simulink model "SIFT-save"  (R2016a)
settings: Solver=VariableStepAuto  StartTime=0.0  StopTime=10.0  RelTol=1e-3
libraries: visionhdlfilter x4, visionhdlio x2, visionsources x1, visiongeotforms x1
settings Model: Creator=Gururaja  LastModifiedBy=Gururaja

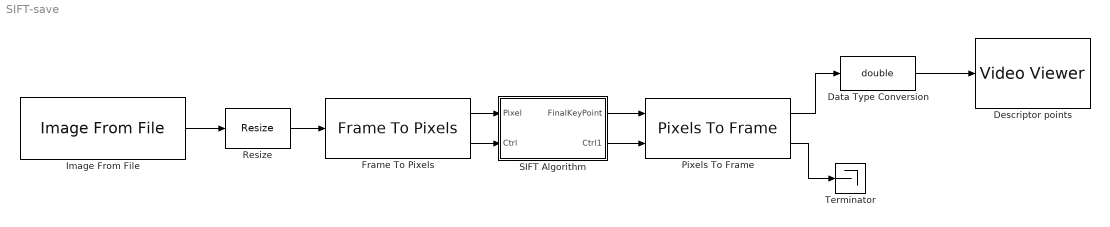
== system SIFT-save ==
  Data Type Conversion : DataTypeConversion  OutDataTypeStr=double
  Descriptor points : VideoViewer
  Frame To Pixels : visionhdlio/Frame To Pixels  NumComponents=1  VideoFormat=1080p  ActivePixelsPerLine=32  ActiveVideoLines=18  TotalPixelsPerLine=42  TotalVideoLines=28  StartingActiveLine=6  FrontPorch=5  SampleTime=0
  Image From File : visionsources/Image From File  Tag=vipblks_nd  FileName=peppers.png  imagePorts=One multidimensional signal  Ts=inf  ImageDataType=Inherit from input image  Signed=on  WordLength=16  sdImageDataType=uint(8)  FractionLengthMode=User-defined  FractionLength=15  OutPortLabels=R|G|B
  Pixels To Frame : visionhdlio/Pixels To Frame  NumComponents=1  VideoFormat=1080p  ActivePixelsPerLine=32  ActiveVideoLines=18  TotalPixelsPerLine=42  TotalVideoLines=28
  Resize : visiongeotforms/Resize  specify=Output size as a percentage of input size  rfactor=[200 150]  outCols=25  outRows=25  outRowsCols=[25 35]  interp_method=Bilinear  antialias=on  useROI=off  roiFlag=off  prodOutputMode=Binary point scaling  prodOutputWordLength=32  prodOutputFracLength=10  roundingMode=Nearest  overflowMode=on
  SIFT Algorithm : Subsystem
  Terminator : Terminator
  wires:
  Image From File/1 -> Resize/1
  Resize/1 -> Frame To Pixels/1
  Frame To Pixels/1 -> SIFT Algorithm/1(Pixel)
  Frame To Pixels/2 -> SIFT Algorithm/2(Ctrl)
  SIFT Algorithm/1(FinalKeyPoint) -> Pixels To Frame/1
  SIFT Algorithm/2(Ctrl1) -> Pixels To Frame/2
  Pixels To Frame/2 -> Terminator/1
  Pixels To Frame/1 -> Data Type Conversion/1
  Data Type Conversion/1 -> Descriptor points/1

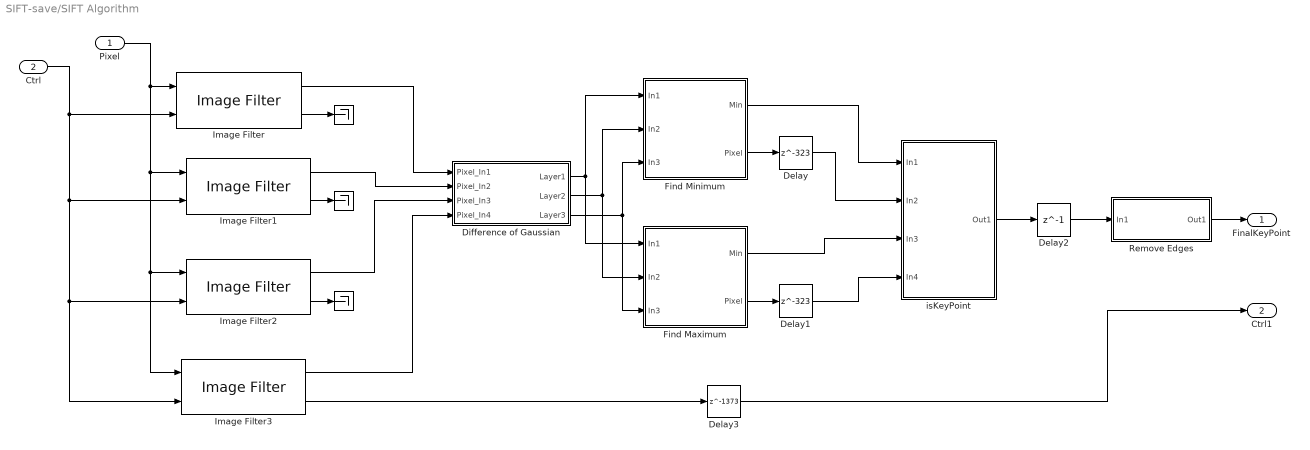
== system SIFT-save/SIFT Algorithm ==
  Pixel : Inport
  Ctrl : Inport  Port=2
  " " : Terminator
  " " : Terminator
  " " : Terminator
  Delay : Delay  DelayLength=323  InitialCondition=0
  Delay1 : Delay  DelayLength=323  InitialCondition=0
  Delay2 : Delay  DelayLength=1  InitialCondition=0
  Delay3 : Delay  DelayLength=1373  InitialCondition=0
  Difference of Gaussian : Subsystem
  Find Maximum : Subsystem
  Find Minimum : Subsystem
  Image Filter{,1..3} (4 alike) : visionhdlfilter/Image Filter  Coefficients=[ 1, 0; 0, -1 ]  PaddingMethod=Constant  PaddingValue=0  LineBufferSize=2048  roundingMode=Floor  overflowMode=off  CoeffMin=[]  CoeffMax=[]  OutputMin=[]  OutputMax=[]  SimulateUsing=Code generation
  Remove Edges : Subsystem
  isKeyPoint : Subsystem
  FinalKeyPoint : Outport
  Ctrl1 : Outport  Port=2
  wires:
  Pixel/1 -> Image Filter/1, Image Filter1/1, Image Filter3/1, Image Filter2/1
  Ctrl/1 -> Image Filter/2, Image Filter1/2, Image Filter2/2, Image Filter3/2
  Image Filter2/2 -> " "/1
  Image Filter1/2 -> " "/1
  Image Filter/2 -> " "/1
  Image Filter/1 -> Difference of Gaussian/1(Pixel_In1)
  Image Filter1/1 -> Difference of Gaussian/2(Pixel_In2)
  Image Filter2/1 -> Difference of Gaussian/3(Pixel_In3)
  Image Filter3/1 -> Difference of Gaussian/4(Pixel_In4)
  Difference of Gaussian/1(Layer1) -> Find Maximum/1(In1), Find Minimum/1(In1)
  Difference of Gaussian/2(Layer2) -> Find Maximum/2(In2), Find Minimum/2(In2)
  Difference of Gaussian/3(Layer3) -> Find Maximum/3(In3), Find Minimum/3(In3)
  Find Minimum/2(Pixel) -> Delay/1
  Find Minimum/1(Min) -> isKeyPoint/1(In1)
  Delay/1 -> isKeyPoint/2(In2)
  Delay1/1 -> isKeyPoint/4(In4)
  isKeyPoint/1(Out1) -> Delay2/1
  Delay2/1 -> Remove Edges/1(In1)
  Remove Edges/1(Out1) -> FinalKeyPoint/1
  Image Filter3/2 -> Delay3/1
  Delay3/1 -> Ctrl1/1
  Find Maximum/1(Min) -> isKeyPoint/3(In3)
  Find Maximum/2(Pixel) -> Delay1/1

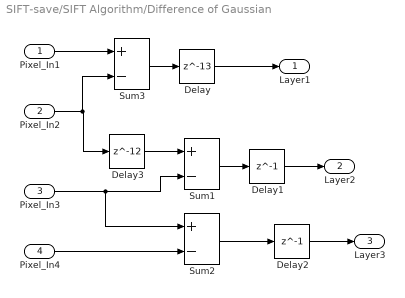
== system SIFT-save/SIFT Algorithm/Difference of Gaussian ==
  Pixel_In1 : Inport
  Pixel_In2 : Inport  Port=2
  Pixel_In3 : Inport  Port=3
  Pixel_In4 : Inport  Port=4
  Delay : Delay  DelayLength=13  InitialCondition=0
  Delay1 : Delay  DelayLength=1  InitialCondition=0
  Delay2 : Delay  DelayLength=1  InitialCondition=0
  Delay3 : Delay  DelayLength=12  InitialCondition=0
  Sum1 : Sum  Inputs=+-
  Sum2 : Sum  Inputs=+-
  Sum3 : Sum  Inputs=+-
  Layer1 : Outport
  Layer2 : Outport  Port=2
  Layer3 : Outport  Port=3
  wires:
  Pixel_In1/1 -> Sum3/1
  Pixel_In2/1 -> Sum3/2, Delay3/1
  Delay3/1 -> Sum1/1
  Pixel_In3/1 -> Sum2/1, Sum1/2
  Pixel_In4/1 -> Sum2/2
  Sum3/1 -> Delay/1
  Sum1/1 -> Delay1/1
  Sum2/1 -> Delay2/1
  Delay2/1 -> Layer3/1
  Delay1/1 -> Layer2/1
  Delay/1 -> Layer1/1

== system SIFT-save/SIFT Algorithm/Find Maximum ==
  In1 : Inport
  In2 : Inport  Port=2
  In3 : Inport  Port=3
  Min/Max DOG1 : Subsystem
  Min/Max DOG2 : Subsystem
  Min/Max DOG3 : Subsystem
  MinMax : MinMax  Function=max  Inputs=26
  Min : Outport
  Pixel : Outport  Port=2
  wires:
  In2/1 -> Min/Max DOG1/1(In1)
  Min/Max DOG1/5(Out5) -> Pixel/1
  Min/Max DOG2/1(Out1) -> MinMax/18
  Min/Max DOG2/9(Out9) -> MinMax/26
  Min/Max DOG2/2(Out2) -> MinMax/19
  Min/Max DOG2/3(Out3) -> MinMax/20
  Min/Max DOG2/4(Out4) -> MinMax/21
  Min/Max DOG2/5(Out5) -> MinMax/22
  Min/Max DOG2/6(Out6) -> MinMax/23
  Min/Max DOG2/7(Out7) -> MinMax/24
  Min/Max DOG2/8(Out8) -> MinMax/25
  Min/Max DOG3/1(Out1) -> MinMax/1
  Min/Max DOG3/3(Out3) -> MinMax/3
  Min/Max DOG3/2(Out2) -> MinMax/2
  Min/Max DOG3/4(Out4) -> MinMax/4
  Min/Max DOG3/5(Out5) -> MinMax/5
  Min/Max DOG3/6(Out6) -> MinMax/6
  Min/Max DOG3/7(Out7) -> MinMax/7
  Min/Max DOG3/8(Out8) -> MinMax/8
  Min/Max DOG3/9(Out9) -> MinMax/9
  MinMax/1 -> Min/1
  Min/Max DOG1/1(Out1) -> MinMax/10
  Min/Max DOG1/2(Out2) -> MinMax/11
  Min/Max DOG1/3(Out3) -> MinMax/12
  Min/Max DOG1/4(Out4) -> MinMax/13
  Min/Max DOG1/6(Out6) -> MinMax/14
  Min/Max DOG1/7(Out7) -> MinMax/15
  Min/Max DOG1/8(Out8) -> MinMax/16
  Min/Max DOG1/9(Out9) -> MinMax/17
  In1/1 -> Min/Max DOG3/1(In1)
  In3/1 -> Min/Max DOG2/1(In1)

== system SIFT-save/SIFT Algorithm/Find Minimum ==
  In1 : Inport
  In2 : Inport  Port=2
  In3 : Inport  Port=3
  Min/Max DOG1 : Subsystem
  Min/Max DOG2 : Subsystem
  Min/Max DOG3 : Subsystem
  MinMax : MinMax  Inputs=26
  Min : Outport
  Pixel : Outport  Port=2
  wires:
  In2/1 -> Min/Max DOG1/1(In1)
  Min/Max DOG1/5(Out5) -> Pixel/1
  Min/Max DOG2/1(Out1) -> MinMax/18
  Min/Max DOG2/9(Out9) -> MinMax/26
  Min/Max DOG2/2(Out2) -> MinMax/19
  Min/Max DOG2/3(Out3) -> MinMax/20
  Min/Max DOG2/4(Out4) -> MinMax/21
  Min/Max DOG2/5(Out5) -> MinMax/22
  Min/Max DOG2/6(Out6) -> MinMax/23
  Min/Max DOG2/7(Out7) -> MinMax/24
  Min/Max DOG2/8(Out8) -> MinMax/25
  Min/Max DOG3/1(Out1) -> MinMax/1
  Min/Max DOG3/3(Out3) -> MinMax/3
  Min/Max DOG3/2(Out2) -> MinMax/2
  Min/Max DOG3/4(Out4) -> MinMax/4
  Min/Max DOG3/5(Out5) -> MinMax/5
  Min/Max DOG3/6(Out6) -> MinMax/6
  Min/Max DOG3/7(Out7) -> MinMax/7
  Min/Max DOG3/8(Out8) -> MinMax/8
  Min/Max DOG3/9(Out9) -> MinMax/9
  MinMax/1 -> Min/1
  Min/Max DOG1/1(Out1) -> MinMax/10
  Min/Max DOG1/2(Out2) -> MinMax/11
  Min/Max DOG1/3(Out3) -> MinMax/12
  Min/Max DOG1/4(Out4) -> MinMax/13
  Min/Max DOG1/6(Out6) -> MinMax/14
  Min/Max DOG1/7(Out7) -> MinMax/15
  Min/Max DOG1/8(Out8) -> MinMax/16
  Min/Max DOG1/9(Out9) -> MinMax/17
  In1/1 -> Min/Max DOG3/1(In1)
  In3/1 -> Min/Max DOG2/1(In1)

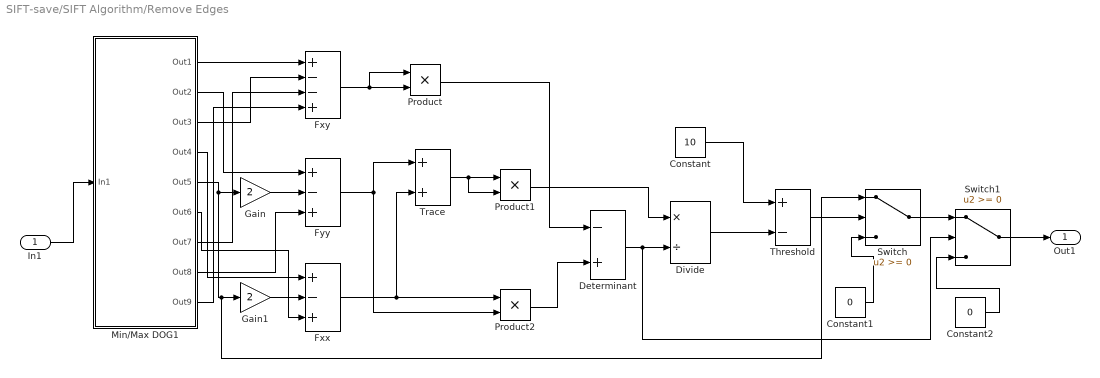
== system SIFT-save/SIFT Algorithm/Remove Edges ==
  In1 : Inport
  Constant : Constant  Value=10
  Constant1 : Constant  Value=0
  Constant2 : Constant  Value=0
  Determinant : Sum  Inputs=-+
  Divide : Product  Inputs=*/
  Fxx : Sum  Inputs=+-+
  Fxy : Sum  Inputs=+--+
  Fyy : Sum  Inputs=+-+
  Gain : Gain  Gain=2
  Gain1 : Gain  Gain=2
  Min/Max DOG1 : Subsystem
  Product : Product
  Product1 : Product
  Product2 : Product
  Switch : Switch
  Switch1 : Switch
  Threshold : Sum  Inputs=+-
  Trace : Sum
  Out1 : Outport
  wires:
  In1/1 -> Min/Max DOG1/1(In1)
  Min/Max DOG1/1(Out1) -> Fxy/1
  Min/Max DOG1/3(Out3) -> Fxy/2
  Gain1/1 -> Fxx/2
  Gain/1 -> Fyy/2
  Min/Max DOG1/2(Out2) -> Fyy/1
  Min/Max DOG1/4(Out4) -> Fxx/1
  Min/Max DOG1/6(Out6) -> Fxx/3
  Min/Max DOG1/7(Out7) -> Fxy/3
  Min/Max DOG1/8(Out8) -> Fyy/3
  Min/Max DOG1/9(Out9) -> Fxy/4
  Fyy/1 -> Product2/2, Trace/1
  Fxy/1 -> Product/1, Product/2
  Trace/1 -> Product1/2, Product1/1
  Fxx/1 -> Trace/2, Product2/1
  Product2/1 -> Determinant/2
  Product/1 -> Determinant/1
  Determinant/1 -> Switch1/2, Divide/2
  Product1/1 -> Divide/1
  Divide/1 -> Threshold/2
  Constant/1 -> Threshold/1
  Threshold/1 -> Switch/2
  Constant1/1 -> Switch/3
  Min/Max DOG1/5(Out5) -> Switch/1, Gain1/1, Gain/1
  Switch/1 -> Switch1/1
  Constant2/1 -> Switch1/3
  Switch1/1 -> Out1/1

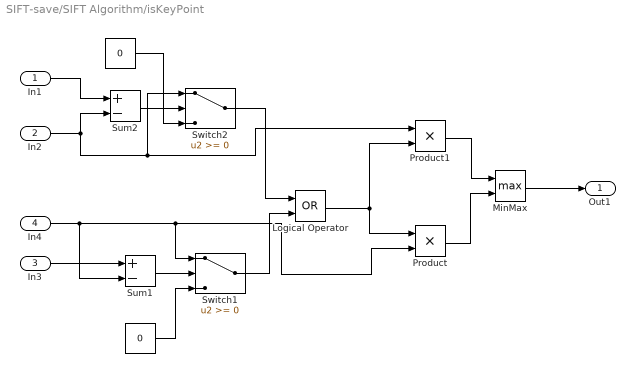
== system SIFT-save/SIFT Algorithm/isKeyPoint ==
  In1 : Inport
  In2 : Inport  Port=2
  In3 : Inport  Port=3
  In4 : Inport  Port=4
  " " : Constant  Value=0
  " " : Constant  Value=0
  Logical Operator : Logic  Operator=OR  AllPortsSameDT=off  OutDataTypeStr=boolean
  MinMax : MinMax  Function=max  Inputs=2
  Product : Product
  Product1 : Product
  Sum1 : Sum  Inputs=+-
  Sum2 : Sum  Inputs=+-
  Switch1 : Switch
  Switch2 : Switch
  Out1 : Outport
  wires:
  In1/1 -> Sum2/1
  In2/1 -> Sum2/2, Switch2/1, Product1/1
  Sum1/1 -> Switch1/2
  Sum2/1 -> Switch2/2
  " "/1 -> Switch2/3
  " "/1 -> Switch1/3
  In3/1 -> Sum1/1
  Switch2/1 -> Logical Operator/1
  Switch1/1 -> Logical Operator/2
  Product1/1 -> MinMax/1
  Product/1 -> MinMax/2
  MinMax/1 -> Out1/1
  Logical Operator/1 -> Product1/2, Product/1
  In4/1 -> Sum1/2, Switch1/1, Product/2

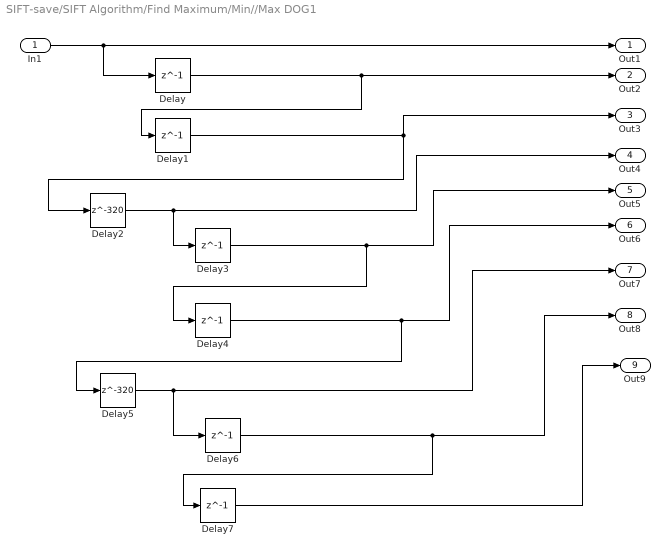
== system SIFT-save/SIFT Algorithm/Find Maximum/Min//Max DOG1 ==
  In1 : Inport
  Delay{,1,3..4,6..7} (6 alike) : Delay  DelayLength=1  InitialCondition=0
  Delay2 : Delay  DelayLength=320  InitialCondition=0
  Delay5 : Delay  DelayLength=320  InitialCondition=0
  Out1 : Outport
  Out2 : Outport  Port=2
  Out3 : Outport  Port=3
  Out4 : Outport  Port=4
  Out5 : Outport  Port=5
  Out6 : Outport  Port=6
  Out7 : Outport  Port=7
  Out8 : Outport  Port=8
  Out9 : Outport  Port=9
  wires:
  In1/1 -> Delay/1, Out1/1
  Delay/1 -> Out2/1, Delay1/1
  Delay1/1 -> Out3/1, Delay2/1
  Delay2/1 -> Delay3/1, Out4/1
  Delay3/1 -> Delay4/1, Out5/1
  Delay4/1 -> Delay5/1, Out6/1
  Delay5/1 -> Delay6/1, Out7/1
  Delay6/1 -> Delay7/1, Out8/1
  Delay7/1 -> Out9/1

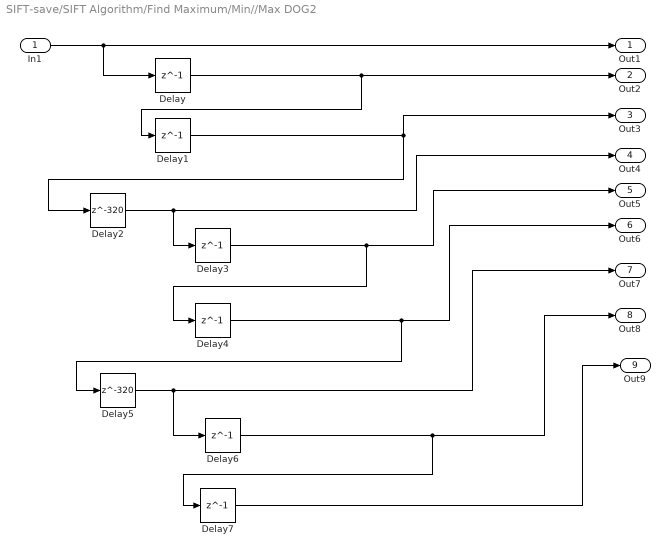
== system SIFT-save/SIFT Algorithm/Find Maximum/Min//Max DOG2 ==
  In1 : Inport
  Delay{,1,3..4,6..7} (6 alike) : Delay  DelayLength=1  InitialCondition=0
  Delay2 : Delay  DelayLength=320  InitialCondition=0
  Delay5 : Delay  DelayLength=320  InitialCondition=0
  Out1 : Outport
  Out2 : Outport  Port=2
  Out3 : Outport  Port=3
  Out4 : Outport  Port=4
  Out5 : Outport  Port=5
  Out6 : Outport  Port=6
  Out7 : Outport  Port=7
  Out8 : Outport  Port=8
  Out9 : Outport  Port=9
  wires:
  In1/1 -> Delay/1, Out1/1
  Delay/1 -> Out2/1, Delay1/1
  Delay1/1 -> Out3/1, Delay2/1
  Delay2/1 -> Delay3/1, Out4/1
  Delay3/1 -> Delay4/1, Out5/1
  Delay4/1 -> Delay5/1, Out6/1
  Delay5/1 -> Delay6/1, Out7/1
  Delay6/1 -> Delay7/1, Out8/1
  Delay7/1 -> Out9/1

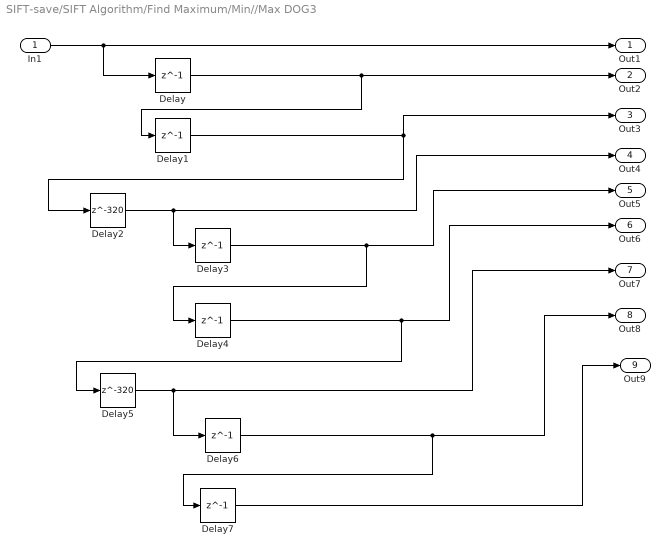
== system SIFT-save/SIFT Algorithm/Find Maximum/Min//Max DOG3 ==
  In1 : Inport
  Delay{,1,3..4,6..7} (6 alike) : Delay  DelayLength=1  InitialCondition=0
  Delay2 : Delay  DelayLength=320  InitialCondition=0
  Delay5 : Delay  DelayLength=320  InitialCondition=0
  Out1 : Outport
  Out2 : Outport  Port=2
  Out3 : Outport  Port=3
  Out4 : Outport  Port=4
  Out5 : Outport  Port=5
  Out6 : Outport  Port=6
  Out7 : Outport  Port=7
  Out8 : Outport  Port=8
  Out9 : Outport  Port=9
  wires:
  In1/1 -> Delay/1, Out1/1
  Delay/1 -> Out2/1, Delay1/1
  Delay1/1 -> Out3/1, Delay2/1
  Delay2/1 -> Delay3/1, Out4/1
  Delay3/1 -> Delay4/1, Out5/1
  Delay4/1 -> Delay5/1, Out6/1
  Delay5/1 -> Delay6/1, Out7/1
  Delay6/1 -> Delay7/1, Out8/1
  Delay7/1 -> Out9/1

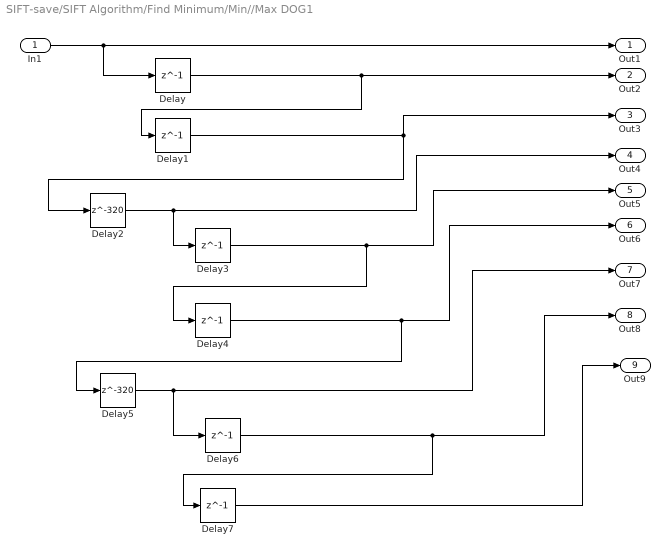
== system SIFT-save/SIFT Algorithm/Find Minimum/Min//Max DOG1 ==
  In1 : Inport
  Delay{,1,3..4,6..7} (6 alike) : Delay  DelayLength=1  InitialCondition=0
  Delay2 : Delay  DelayLength=320  InitialCondition=0
  Delay5 : Delay  DelayLength=320  InitialCondition=0
  Out1 : Outport
  Out2 : Outport  Port=2
  Out3 : Outport  Port=3
  Out4 : Outport  Port=4
  Out5 : Outport  Port=5
  Out6 : Outport  Port=6
  Out7 : Outport  Port=7
  Out8 : Outport  Port=8
  Out9 : Outport  Port=9
  wires:
  In1/1 -> Delay/1, Out1/1
  Delay/1 -> Out2/1, Delay1/1
  Delay1/1 -> Out3/1, Delay2/1
  Delay2/1 -> Delay3/1, Out4/1
  Delay3/1 -> Delay4/1, Out5/1
  Delay4/1 -> Delay5/1, Out6/1
  Delay5/1 -> Delay6/1, Out7/1
  Delay6/1 -> Delay7/1, Out8/1
  Delay7/1 -> Out9/1

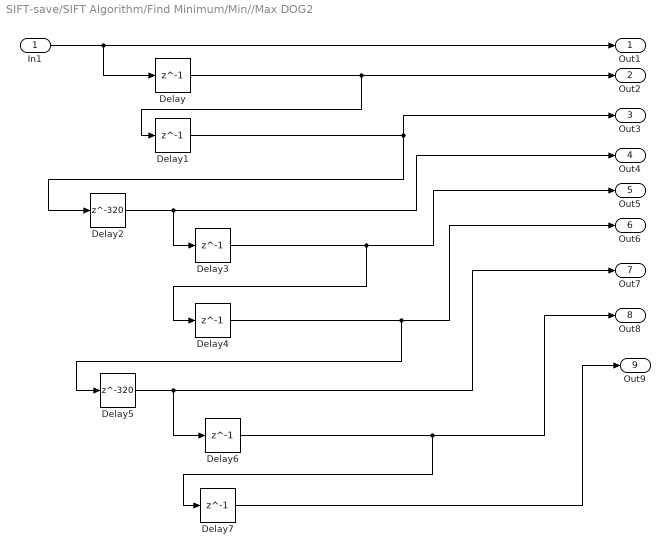
== system SIFT-save/SIFT Algorithm/Find Minimum/Min//Max DOG2 ==
  In1 : Inport
  Delay{,1,3..4,6..7} (6 alike) : Delay  DelayLength=1  InitialCondition=0
  Delay2 : Delay  DelayLength=320  InitialCondition=0
  Delay5 : Delay  DelayLength=320  InitialCondition=0
  Out1 : Outport
  Out2 : Outport  Port=2
  Out3 : Outport  Port=3
  Out4 : Outport  Port=4
  Out5 : Outport  Port=5
  Out6 : Outport  Port=6
  Out7 : Outport  Port=7
  Out8 : Outport  Port=8
  Out9 : Outport  Port=9
  wires:
  In1/1 -> Delay/1, Out1/1
  Delay/1 -> Out2/1, Delay1/1
  Delay1/1 -> Out3/1, Delay2/1
  Delay2/1 -> Delay3/1, Out4/1
  Delay3/1 -> Delay4/1, Out5/1
  Delay4/1 -> Delay5/1, Out6/1
  Delay5/1 -> Delay6/1, Out7/1
  Delay6/1 -> Delay7/1, Out8/1
  Delay7/1 -> Out9/1

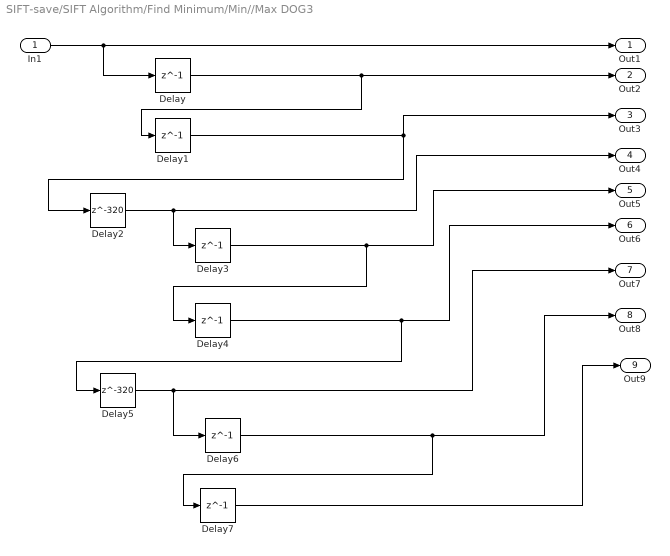
== system SIFT-save/SIFT Algorithm/Find Minimum/Min//Max DOG3 ==
  In1 : Inport
  Delay{,1,3..4,6..7} (6 alike) : Delay  DelayLength=1  InitialCondition=0
  Delay2 : Delay  DelayLength=320  InitialCondition=0
  Delay5 : Delay  DelayLength=320  InitialCondition=0
  Out1 : Outport
  Out2 : Outport  Port=2
  Out3 : Outport  Port=3
  Out4 : Outport  Port=4
  Out5 : Outport  Port=5
  Out6 : Outport  Port=6
  Out7 : Outport  Port=7
  Out8 : Outport  Port=8
  Out9 : Outport  Port=9
  wires:
  In1/1 -> Delay/1, Out1/1
  Delay/1 -> Out2/1, Delay1/1
  Delay1/1 -> Out3/1, Delay2/1
  Delay2/1 -> Delay3/1, Out4/1
  Delay3/1 -> Delay4/1, Out5/1
  Delay4/1 -> Delay5/1, Out6/1
  Delay5/1 -> Delay6/1, Out7/1
  Delay6/1 -> Delay7/1, Out8/1
  Delay7/1 -> Out9/1

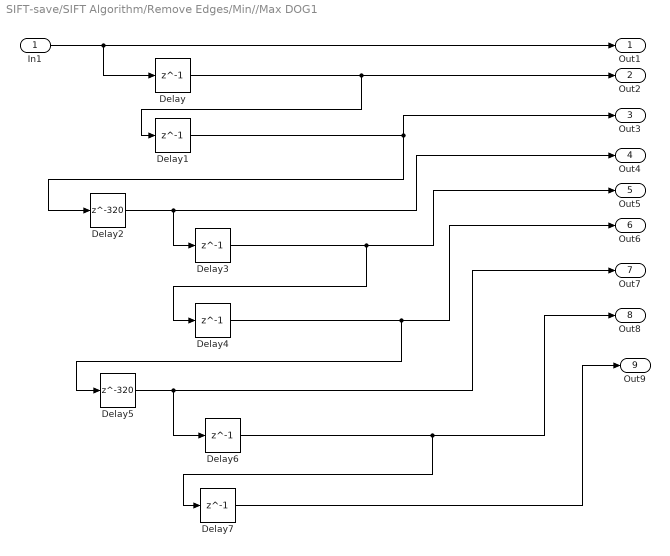
== system SIFT-save/SIFT Algorithm/Remove Edges/Min//Max DOG1 ==
  In1 : Inport
  Delay{,1,3..4,6..7} (6 alike) : Delay  DelayLength=1  InitialCondition=0
  Delay2 : Delay  DelayLength=320  InitialCondition=0
  Delay5 : Delay  DelayLength=320  InitialCondition=0
  Out1 : Outport
  Out2 : Outport  Port=2
  Out3 : Outport  Port=3
  Out4 : Outport  Port=4
  Out5 : Outport  Port=5
  Out6 : Outport  Port=6
  Out7 : Outport  Port=7
  Out8 : Outport  Port=8
  Out9 : Outport  Port=9
  wires:
  In1/1 -> Delay/1, Out1/1
  Delay/1 -> Out2/1, Delay1/1
  Delay1/1 -> Out3/1, Delay2/1
  Delay2/1 -> Delay3/1, Out4/1
  Delay3/1 -> Delay4/1, Out5/1
  Delay4/1 -> Delay5/1, Out6/1
  Delay5/1 -> Delay6/1, Out7/1
  Delay6/1 -> Delay7/1, Out8/1
  Delay7/1 -> Out9/1
